simulink model "Ejercicio_2_DB"  (R2023a)
settings: Solver=VariableStepAuto  StartTime=0.0  StopTime=10  RelTol=1e-3
values from neighbouring files (symbols this model uses):
  g0 = 1/(C_ss*inv(-A_ss+B_ss*K_ss)*B_ss)    [Ejercicio_1_c.m]
  K_ss = acker(A_ss,B_ss,PLC)    [Ejercicio_1_c.m]
undefined symbols (not defined in the file or in its folder): A_ss, B_ss, C_ss, D_ss
settings Model: Creator=Mati  LastModifiedBy=Mati

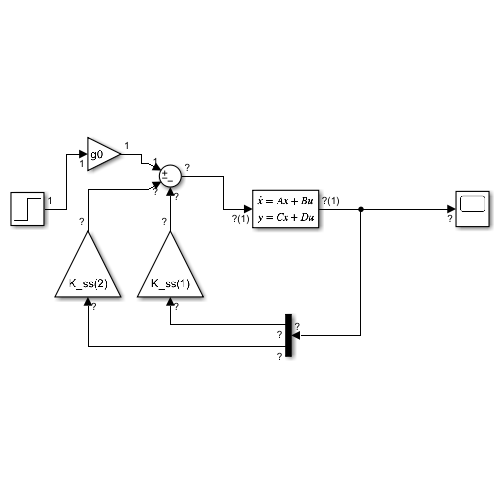
[thumbnail: Simulink's stored preview of the top-level diagram]
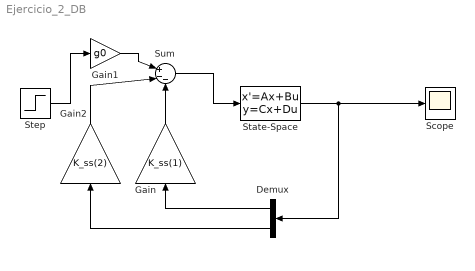
== system Ejercicio_2_DB ==
  Demux : Demux  Outputs=2
  Gain : Gain  Gain=K_ss(1)
  Gain1 : Gain  Gain=g0
  Gain2 : Gain  Gain=K_ss(2)
  Scope : Scope
  State-Space : StateSpace  A=A_ss  B=B_ss  C=C_ss  D=D_ss  InitialCondition=0  ContinuousStateAttributes='654'
  Step : Step  SampleTime=0
  Sum : Sum  Inputs=|+--
  wires:
  Sum/1 -> State-Space/1
  State-Space/1 -> Scope/1, Demux/1
  Gain/1 -> Sum/3
  Step/1 -> Gain1/1
  Gain1/1 -> Sum/1
  Demux/1 -> Gain/1
  Demux/2 -> Gain2/1
  Gain2/1 -> Sum/2
